simulink model "tp403264"  (Simulink 3.0)
settings: Solver=ode1  SolverMode=SingleTasking  StartTime=0.0  StopTime=t_sim  FixedStep=Ts  RelTol=1e-3
values from neighbouring files (symbols this model uses):
  Ks = input('Put integrator gain value Ks = ')    [init_PI1_windupless.m]    (also in init_PID1_windupless_tune3.m)
  P = input('Put gain of P component = ')    [init_PI1_windupless.m]    (also in init_PID1_windupless_tune3.m; init_step_resp2.m = 2)
  Ts = 1    [init_PI1_windupless.m]    (also in init_PID1_windupless_tune3.m = 0.5; init_step_resp2.m = 0.2; prev45_0.mat = 0.2; prev45_1.mat = 0.2)
  Umax = 5    [init_PI1_windupless.m]    (also in init_PID1_windupless_tune3.m; init_step_resp2.m; prev45_0.mat; prev45_1.mat)
  Umin = 0    [init_PI1_windupless.m]    (also in init_PID1_windupless_tune3.m; init_step_resp2.m; prev45_0.mat; prev45_1.mat)
  y0 = mean(yt(t_prep_in-10:t_prep_in,3))    [init_step_resp2.m]
undefined symbols (not defined in the file or in its folder): a, D, filt0, Ka, lambda
libraries: simulink x1, udaq28LT_lib x1
settings Model: LastModifiedBy=mato  ExtModeMexFile=rtwinext  ExtModeTrigDuration=100000  SaveFormat=Matrix  RTWSystemTargetFile=rtwin.tlc  RTWTemplateMakefile=rtwintmf  RTWOptions="-aCCOptimize=1 -aEnforceIntegerDowncast=1 -aExtMode=1 -aFoldNonRolledExpr=1 -aForceParamTrailComments=0 -aGenerateComments=1 -aGenerateReport=0 -aIncDataTypeInIds=0 -aIncHierarchyInIds=0 -aInlineInvariantSignals=0 -aInlinedPrmAccess=\"Literals\" -aLocalBlockOutputs=1 -aMaxRTWIdLen=31 -aPrefixModelToSubsysFcnNames=1 -aRTWVerbose=1 -aRebuildAll=1 -aRollThreshold=5 -aShowEliminatedStatements=1"

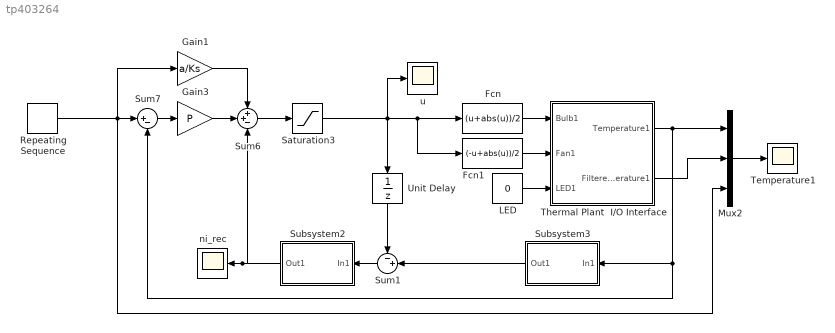
== system tp403264 ==
  Fcn : Fcn  Expr=(u+abs(u))/2
  Fcn1 : Fcn  Expr=(-u+abs(u))/2
  Gain1 : Gain  Gain=a/Ks  SaturateOnIntegerOverflow=on
  Gain3 : Gain  Gain=P  SaturateOnIntegerOverflow=on
  LED : Constant  Value=0
  Mux2 : Mux  Inputs=3
  Repeating Sequence : simulink/Sources/Repeating Sequence  rep_seq_t=[0 180 180 430 430 600]  rep_seq_y=[y0+3 y0+3 y0+5 y0+5 y0+3 y0+3 ]
  Saturation3 : Saturate  UpperLimit=Umax  LowerLimit=Umin
  Subsystem2 : Subsystem  Orientation=left
  Subsystem3 : Subsystem  Orientation=left
  Sum1 : Sum  Orientation=left  Inputs=-+|  SaturateOnIntegerOverflow=on
  Sum6 : Sum  Inputs=++-  SaturateOnIntegerOverflow=on
  Sum7 : Sum  Inputs=|+-  SaturateOnIntegerOverflow=on
  Temperature1 : Scope
      settings: TickLabels=on  TimeRange=30  YMin=27  YMax=34  SaveName=yt  DataFormat=Matrix
  Thermal Plant  I/O Interface : Subsystem
      mask Display: disp('Thermo-optical\nPlant\nI/O Interface')
  Unit Delay : UnitDelay  Orientation=down  X0=0  SampleTime=Ts
  ni_rec : Scope
      settings: TimeRange=auto  YMin=-0.5  YMax=1.1  SaveName=ni_rec  DataFormat=Matrix  Decimation=10  SampleInput=on  SampleTime=Ts
  u : Scope
      settings: TimeRange=80  YMin=1.925  YMax=2.425  SaveName=u  DataFormat=Matrix  Decimation=10  SampleInput=on  SampleTime=Ts
  wires:
  Unit Delay/1 -> Sum1/1
  Subsystem3/1(Out1) -> Sum1/2
  Sum6/1 -> Saturation3/1
  Saturation3/1 -> u/1, Unit Delay/1, Fcn1/1, Fcn/1
  Repeating Sequence/1 -> Sum7/1, Gain1/1, Mux2/3
  Sum7/1 -> Gain3/1
  Sum1/1 -> Subsystem2/1(In1)
  Subsystem2/1(Out1) -> Sum6/3, ni_rec/1
  Gain1/1 -> Sum6/1
  Gain3/1 -> Sum6/2
  Mux2/1 -> Temperature1/1
  Fcn/1 -> Thermal Plant  I/O Interface/1(Bulb1)
  Fcn1/1 -> Thermal Plant  I/O Interface/2(Fan1)
  LED/1 -> Thermal Plant  I/O Interface/3(LED1)
  Thermal Plant  I/O Interface/1(Temperature1) -> Mux2/1, Subsystem3/1(In1), Sum7/2
  Thermal Plant  I/O Interface/2(Filtered  temperature1) -> Mux2/2

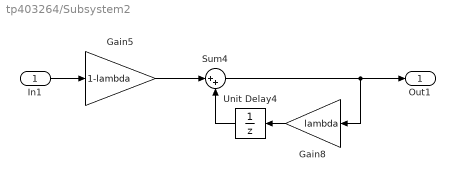
== system tp403264/Subsystem2 ==
  In1 : Inport  Port=1  PortWidth=-1  SampleTime=-1  DataType=auto
      settings: SignalType=auto
  Gain5 : Gain  Gain=1-lambda  SaturateOnIntegerOverflow=on
  Gain8 : Gain  Orientation=left  Gain=lambda  SaturateOnIntegerOverflow=on
  Sum4 : Sum  Inputs=|++  SaturateOnIntegerOverflow=on
  Unit Delay4 : UnitDelay  Orientation=left  X0=filt0  SampleTime=Ts
  Out1 : Outport  Port=1
  wires:
  Gain5/1 -> Sum4/1
  Sum4/1 -> Gain8/1, Out1/1
  Gain8/1 -> Unit Delay4/1
  Unit Delay4/1 -> Sum4/2
  In1/1 -> Gain5/1

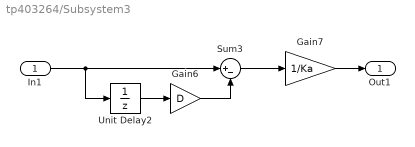
== system tp403264/Subsystem3 ==
  In1 : Inport  Port=1  PortWidth=-1  SampleTime=-1  DataType=auto
      settings: SignalType=auto
  Gain6 : Gain  Gain=D  SaturateOnIntegerOverflow=on
  Gain7 : Gain  Gain=1/Ka  SaturateOnIntegerOverflow=on
  Sum3 : Sum  Inputs=|+-  SaturateOnIntegerOverflow=on
  Unit Delay2 : UnitDelay  X0=y0  SampleTime=Ts
  Out1 : Outport  Port=1
  wires:
  Gain7/1 -> Out1/1
  Unit Delay2/1 -> Gain6/1
  In1/1 -> Unit Delay2/1, Sum3/1
  Gain6/1 -> Sum3/2
  Sum3/1 -> Gain7/1

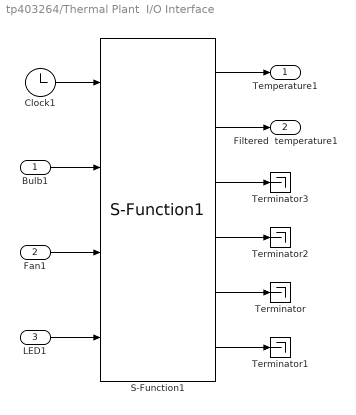
== system tp403264/Thermal Plant  I/O Interface ==
  Bulb1 : Inport  Port=1  PortWidth=-1  SampleTime=-1  DataType=auto
      settings: SignalType=auto
  Fan1 : Inport  Port=2  PortWidth=-1  SampleTime=-1  DataType=auto
      settings: SignalType=auto
  LED1 : Inport  Port=3  PortWidth=-1  SampleTime=-1  DataType=auto
      settings: SignalType=auto
  Clock1 : Clock
      settings: DisplayTime=off  Decimation=10
  S-Function1 : udaq28LT_lib/S-Function1  Priority=1  com_port=COM3  Ts=Ts  events_ot=2  rd_timeout=Ts/2*1000  matlab_prior=ABOVE_NORMAL_PRIORITY  warning=on  printout=off
  Terminator{,1..3} (4 alike) : Terminator
  Temperature1 : Outport  Port=1
  Filtered  temperature1 : Outport  Port=2
  wires:
  S-Function1/1 -> Temperature1/1
  S-Function1/2 -> Filtered  temperature1/1
  Clock1/1 -> S-Function1/1
  Bulb1/1 -> S-Function1/2
  Fan1/1 -> S-Function1/3
  S-Function1/3 -> Terminator3/1
  S-Function1/4 -> Terminator2/1
  S-Function1/5 -> Terminator/1
  S-Function1/6 -> Terminator1/1
  LED1/1 -> S-Function1/4
